simulink model "Ball_balancing_platform_Multibody_FINAL"  (R2020b)
settings: Solver=VariableStepAuto  StartTime=0.0  StopTime=15  RelTol=1e-4  AbsTol=0.1  EnableMultiTasking=on
model workspace (MAT data in the model file):
  Amplitude = 0.02
  amp = 0
  var = 0.02
undefined symbols (not defined in the file): X, Y, Z
libraries: sm_lib x23, fl_lib x16, nesl_utility x13, ee_lib x2
(part 2 of 2)

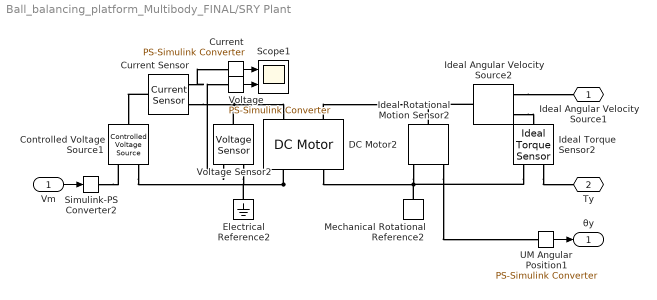
== system Ball_balancing_platform_Multibody_FINAL/SRY Plant ==
  Vm : Inport
  Controlled Voltage Source1 : fl_lib/Electrical/Electrical Sources/Controlled Voltage Source
  Current : nesl_utility/PS-Simulink Converter  PhysicalDomain=network_engine_domain  SubClassName=ps_output  LeftPortType=input  RightPortType=output  PseudoPeriodic=off  Frequencies=[]  Unit=inherit  AffineConversion=off
  Current Sensor : fl_lib/Electrical/Electrical Sensors/Current Sensor
  DC Motor2 : ee_lib/Electromechanical/Brushed Motors/DC Motor  field_option=ee.enum.field_option.pm  Rf=100 Ohm  Lf=1 H  Laf=0.15 H  If0=0 A  parameterization=ee.enum.dcparam_option.circuit_param  Ra=0.7 Ohm  La=0.5 mH  emf_or_torque=ee.enum.emf_or_torque.kv  Kv=0.0342 V/(rad/s)  Ki=242 N*m/A  T_stall=0.24e-3 N*m  w_max=19100 rpm  w_rated=15000 rpm  P_rated=0.08 W  V_rated=1.5 V  J=282.5 g*cm^2  lam_param=ee.enum.lam_param.damping  lam=0 N*m/(rad/s)  i_noload=0 A  V_i_noload=1.5 V  speed0=0 rpm  enable_fault_armature=ee.enum.faults.faultEnable.no  rev_faulted=1 / 3  G_faulted_armature=1e-5 S  fault_trigger_armature=ee.enum.faults.faultTrigger.temporal  t_fault_armature=1 s  max_permissible_current_armature=inf A  t_fail_on_current_armature=1 s  enable_fault_field=ee.enum.faults.faultEnable.no  G_faulted_field=1e-5 S  fault_trigger_field=ee.enum.faults.faultTrigger.temporal  t_fault_field=1 s  max_permissible_current_field=inf A  t_fail_on_current_field=1 s  fault_action=ee.enum.faults.faultAction.none  alpha=3.93e-3 1/K  Tmeas=25 degC  thermal_mass=100 J/K  initial_temperature=25 degC
  Electrical Reference2 : fl_lib/Electrical/Electrical Elements/Electrical Reference
  Ideal Angular Velocity Source2 : fl_lib/Mechanical/Mechanical Sources/Ideal Angular Velocity Source
  Ideal Rotational Motion Sensor2 : fl_lib/Mechanical/Mechanical Sensors/Ideal Rotational Motion Sensor  wrap_angle=simscape.enum.onoff.off  offset=0 rad
  Ideal Torque Sensor2 : fl_lib/Mechanical/Mechanical Sensors/Ideal Torque Sensor
  Mechanical Rotational Reference2 : fl_lib/Mechanical/Rotational Elements/Mechanical Rotational Reference
  Scope1 : Scope  NumInputPorts=2
  Simulink-PS Converter2 : nesl_utility/Simulink-PS Converter  PhysicalDomain=network_engine_domain  SubClassName=ps_input  LeftPortType=input  RightPortType=output  PseudoPeriodic=off  Frequencies=[]  NoiseDistribution=none  NoiseParameters=[]  Unit=1  AffineConversion=off  FilteringAndDerivatives=provide  SimscapeFilterOrder=1  InputFilterTimeConstant=0.001  UdotUserProvided=0
  UM Angular Position1 : nesl_utility/PS-Simulink Converter  PhysicalDomain=network_engine_domain  SubClassName=ps_output  LeftPortType=input  RightPortType=output  PseudoPeriodic=off  Frequencies=[]  Unit=inherit  AffineConversion=off
  Voltage : nesl_utility/PS-Simulink Converter  PhysicalDomain=network_engine_domain  SubClassName=ps_output  LeftPortType=input  RightPortType=output  PseudoPeriodic=off  Frequencies=[]  Unit=inherit  AffineConversion=off
  Voltage Sensor2 : fl_lib/Electrical/Electrical Sensors/Voltage Sensor
  Ideal Angular Velocity Source1 : PMIOPort  Side=Right
  Ty : PMIOPort  Port=2  Side=Right
  θy : Outport
  wires:
  Vm/1 -> Simulink-PS Converter2/1
  UM Angular Position1/1 -> θy/1
  Current/1 -> Scope1/1
  Voltage/1 -> Scope1/2
  connections:
  Ideal Angular Velocity Source2/LConn1 -- DC Motor2/LConn2 -- Ideal Rotational Motion Sensor2/LConn1
  Ideal Rotational Motion Sensor2/RConn3 -- UM Angular Position1/LConn1
  Voltage Sensor2/LConn1 -- Current Sensor/RConn2 -- DC Motor2/LConn1
  Ideal Torque Sensor2/RConn2 -- Ty/RConn1
  Ideal Torque Sensor2/RConn1 -- Ideal Rotational Motion Sensor2/RConn1 -- DC Motor2/RConn2 -- Mechanical Rotational Reference2/LConn1
  Ideal Angular Velocity Source2/RConn2 -- Ideal Torque Sensor2/LConn1
  DC Motor2/RConn1 -- Controlled Voltage Source1/RConn2 -- Voltage Sensor2/RConn2 -- Electrical Reference2/LConn1
  Simulink-PS Converter2/RConn1 -- Controlled Voltage Source1/RConn1
  Ideal Angular Velocity Source2/RConn1 -- Ideal Angular Velocity Source1/RConn1
  Current Sensor/RConn1 -- Current/LConn1
  Current Sensor/LConn1 -- Controlled Voltage Source1/LConn1
  Voltage Sensor2/RConn1 -- Voltage/LConn1

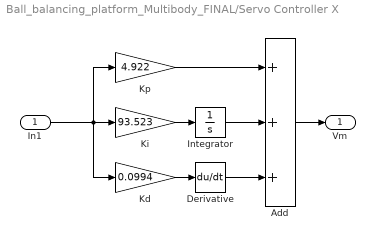
== system Ball_balancing_platform_Multibody_FINAL/Servo Controller X ==
  In1 : Inport
  Add : Sum  Inputs=+++
  Derivative : Derivative
  Integrator : Integrator
  Kd : Gain  Gain=0.0994
  Ki : Gain  Gain=93.523
  Kp : Gain  Gain=4.922
  Vm : Outport
  wires:
  In1/1 -> Kp/1, Kd/1, Ki/1
  Derivative/1 -> Add/3
  Integrator/1 -> Add/2
  Kd/1 -> Derivative/1
  Kp/1 -> Add/1
  Add/1 -> Vm/1
  Ki/1 -> Integrator/1

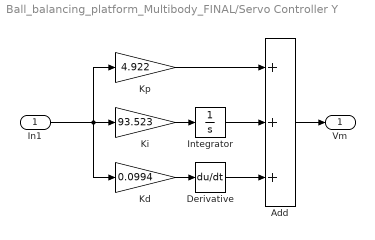
== system Ball_balancing_platform_Multibody_FINAL/Servo Controller Y ==
  In1 : Inport
  Add : Sum  Inputs=+++
  Derivative : Derivative
  Integrator : Integrator
  Kd : Gain  Gain=0.0994
  Ki : Gain  Gain=93.523
  Kp : Gain  Gain=4.922
  Vm : Outport
  wires:
  Ki/1 -> Integrator/1
  Add/1 -> Vm/1
  Kp/1 -> Add/1
  Kd/1 -> Derivative/1
  Integrator/1 -> Add/2
  Derivative/1 -> Add/3
  In1/1 -> Ki/1, Kd/1, Kp/1
